simulink model "Bicycle_Posture_Regulator"  (R2024b)
settings: Solver=ode45  StartTime=0.0  StopTime=40  RelTol=1e-5
libraries: robotmobilelib x1, sim3dlib x1, sim3dautolib x1
settings Model: Creator=loren  LastModifiedBy=loren

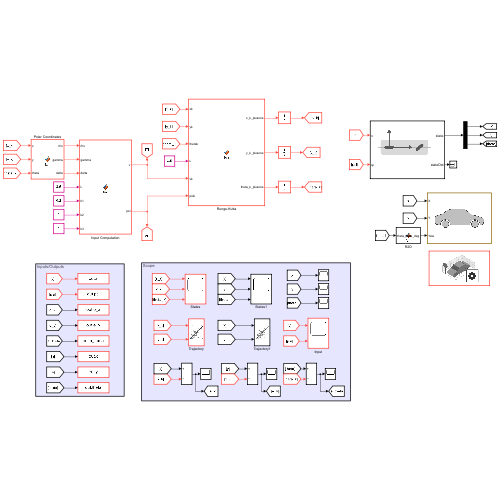
[thumbnail: Simulink's stored preview of the top-level diagram]
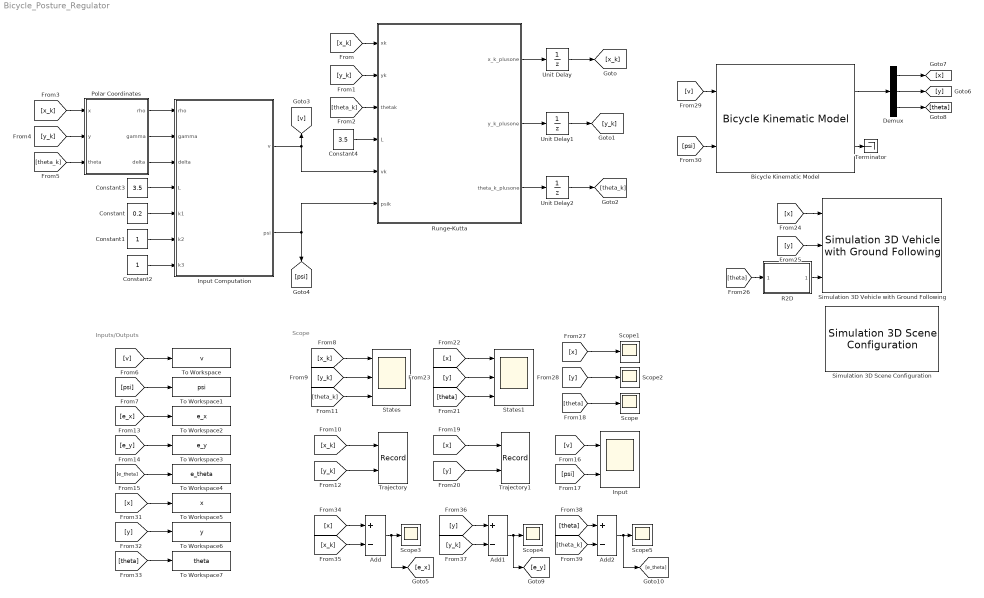
== system Bicycle_Posture_Regulator ==
  note: Scope
  note: Inputs/Outputs
  Add : Sum  Inputs=+-
  Add1 : Sum  Inputs=+-
  Add2 : Sum  Inputs=+-
  Bicycle Kinematic Model : robotmobilelib/Bicycle Kinematic Model  VehicleInputs=Vehicle Speed & Steering Angle  WheelBase=3.5  VehicleSpeedRange=[-inf inf]  MaxSteeringAngle=pi/3  InitialState=[-100; -50; pi/4]  SimulateUsing=Interpreted execution
  Constant : Constant  Value=0.2
  Constant1 : Constant
  Constant2 : Constant
  Constant3 : Constant  Value=3.5
  Constant4 : Constant  Value=3.5
  Demux : Demux  Outputs=3
  Input : Scope  NumInputPorts=2
  Input Computation : MATLAB Function  TreatAsAtomicUnit=on
  Polar Coordinates : MATLAB Function  TreatAsAtomicUnit=on
  R2D : MATLAB Function  TreatAsAtomicUnit=on
  Runge-Kutta : MATLAB Function  TreatAsAtomicUnit=on
  Scope{,1..5} (6 alike) : Scope
  Simulation 3D Scene Configuration : sim3dlib/Simulation 3D Scene Configuration  Priority=0  ProjectFormat=Default Scenes  SceneDesc=Parking lot  ProjectName=C:\Program Files\MATLAB\R2024b\toolbox\shared\sim3d_projects\automotive_project_windows\UE\WindowsNoEditor\VehicleSimulation.exe  ScenePath=/Game/Maps/HwStrght  EnableOpenDRIVE=off  vehTagList={'Custom';'Scene Origin';'SimulinkVehicle1'}  vehTag=SimulinkVehicle1  FreeCameraInitialTranslation=[0, 0, 0]  FreeCameraDefaultInitialTranslation=[-6, 0, 2]  FreeCameraInitialRotation=[0, 0, 0]  FreeCameraDefaultInitialRotation=[0, -15, 0]  OpVisEn=off  Ts=0.01  EnableWindow=on  EnableRemoteAccess=off  EnableWeather=off  SunAzimuth=90  SunAltitude=40.0  EnableGeospatialSun=off  Latitude=0  Longitude=0  Date=2023-01-01  Time=10:30:00  GeoTimeZone=-5.0  SunDaylightSaving=off  wind=1  clouds=10  EnableVolumetricClouds=off  CloudCoverage=0  CloudAltitude=6  fog=0  rain=0  RaindropsEffect=off  SnowDensity=0  EnableGeospatial=off  UseTrueOrigin=off  OriginHeight=200  OriginLatitude=40.744652  OriginLongitude=-73.988864  MapStyle=Aerial  AdditionalAssetIDs=[]  UseAdvancedSunSky=off  SolarTime=11  TimeZone=-5  Day=21  Month=9  Year=2022  UseDaylightSavingTime=on  DSTStartDay=10  DSTStartMonth=3  DSTEndDay=3  DSTEndMonth=11  DSTSwitchHour=2  sensorTag=MainCamera1  sensorId=1  sensorName=MainCamera1  mountLoc=Origin  offsetFlag=off  tmountOffset=[0, 0, 0]  rmountOffset=[0, 0, 0]  HorizontalResolution=1280  VerticalResolution=720  HorizontalFOV=60  mountPoint=[0 0 0]  mountOrientation=[0 0 0]  aMode=3  ID=1  GeoTrigger=Inactive
      settings: LibrarySourceBlock=drivingsim3d/Simulation 3D Scene Configuration
  Simulation 3D Vehicle with Ground Following : sim3dautolib/Simulation 3D Vehicle with Ground Following  Priority=-1  PassVehMesh=Muscle car  MeshPath=/MathWorksAutomotiveContent/Vehicles/Muscle/Meshes/SK_MuscleCar.SK_MuscleCar  TrackWidth=1.9  WheelBase=3  WheelRadius=0.35  VehColor=Red  InitialPos=[-100, -50, 0]  InitialRot=[0, 0, pi/4]  ActorName=SimulinkVehicle1  SampleTime=0.01  ActorType=SimulinkVehicle  ID=1  aMode=3  ActorTag=SimulinkVehicle1  CoordinateScheme=ISO  VehLightsControl=off  HeadlightColor=[ 1, 1, 1 ]  HighBeamIntensity=100000  LowBeamIntensity=60000  HighBeamConeAngle=70  LowBeamConeAngle=70  LeftHeadlightOrientation=[ 0, 0 ]  RightHeadlightOrientation=[ 0, 0 ]  BrakelightIntensity=500  ReverselightIntensity=500  SignallightIntensity=500  SignallightPeriod=1  SignalPulseWidth=50  TransformOutportEnabled=off
      settings: LibrarySourceBlock=drivingsim3d/Simulation 3D Vehicle with Ground Following
  States : Scope  NumInputPorts=3
  States1 : Scope  NumInputPorts=3
  Terminator : Terminator
  To Workspace : ToWorkspace  VariableName=v  SaveFormat=Timeseries  SampleTime=0.01
  To Workspace1 : ToWorkspace  VariableName=psi  SaveFormat=Timeseries  SampleTime=0.01
  To Workspace2 : ToWorkspace  VariableName=e_x  SaveFormat=Timeseries  SampleTime=0.01
  To Workspace3 : ToWorkspace  VariableName=e_y  SaveFormat=Timeseries  SampleTime=0.01
  To Workspace4 : ToWorkspace  VariableName=e_theta  SaveFormat=Timeseries  SampleTime=0.01
  To Workspace5 : ToWorkspace  VariableName=x  SaveFormat=Timeseries  SampleTime=0.01
  To Workspace6 : ToWorkspace  VariableName=y  SaveFormat=Timeseries  SampleTime=0.01
  To Workspace7 : ToWorkspace  VariableName=theta  SaveFormat=Timeseries  SampleTime=0.01
  Trajectory : Record  FileSettingsInternal="{\"entries\":[{\"content\":{\"excelSettings\":{\"content\":{},\"type\":\"Streamout.ExcelSettings\"}},\"type\":\"Streamout.FileSettingStorage\",\"uuid\":\"\"}],\"packageUris\":[\"http:\\/\\/schema.mathworks.com\\/mf0\\/streamout_blocks\\/R2020a\"],\"version\":\"1.0\"}"  Layout=[1 1]  SignalsInternal="{\"entries\":[{\"content\":{\"signals\":[{\"content\":{\"blockPath\":[],\"dimensions\":[1],\"domain\":\"\",\"lineColor\":\"#fe330a\",\"lineWidth\":2,\"port\":1,\"sid\":[\"\"],\"signalID\":1,\"signalName\":\"From10\"},\"type\":\"RecordBlkView.Signal\",\"uuid\":\"\"},{\"content\":{\"blockPath\":[],\"dimensions\":[1],\"domain\":\"\",\"lineColor\":\"#22b573\",\"lineWidth\":2,\"port\":2,\"sid\":[\"\"],\"signalID\":2,\"signalName\":\"From12\"},\"type\":\"RecordBlkView.Signal\",\"uuid\":\"\"}]},\"type\":\"RecordBlkView.InputSignals\",\"uuid\":\"\"}],\"packageUris\":[\"http:\\/\\/schema.mathworks.com\\/mf0\\/streamout_blocks\\/R2020a\"],\"version\":\"1.0\"}"  VisualizationBindings="{\"xyplotplugin\":{\"info\":[{\"series\":[],\"subplotID\":1}]}}"  CompatibilityTag=XY
  Trajectory1 : Record  FileSettingsInternal="{\"entries\":[{\"content\":{\"excelSettings\":{\"content\":{},\"type\":\"Streamout.ExcelSettings\"}},\"type\":\"Streamout.FileSettingStorage\",\"uuid\":\"\"}],\"packageUris\":[\"http:\\/\\/schema.mathworks.com\\/mf0\\/streamout_blocks\\/R2020a\"],\"version\":\"1.0\"}"  Layout=[1 1]  SignalsInternal="{\"entries\":[{\"content\":{\"signals\":[{\"content\":{\"blockPath\":[],\"dimensions\":[1],\"domain\":\"\",\"lineColor\":\"#a2142f\",\"plots\":[ 1 ],\"port\":1,\"sid\":[\"\"],\"signalID\":1,\"signalName\":\"From19\"},\"type\":\"RecordBlkView.Signal\",\"uuid\":\"\"},{\"content\":{\"blockPath\":[],\"dimensions\":[1],\"domain\":\"\",\"lineColor\":\"#139fff\",\"plots\":[ 1 ],\"port\":2,\"sid\":[\"\"],\"signalID\":2,\"signalName\":\"From20\"},\"type\":\"RecordBlkView.Signal\",\"uuid\":\"\"}]},\"type\":\"RecordBlkView.InputSignals\",\"uuid\":\"\"}],\"packageUris\":[\"http:\\/\\/schema.mathworks.com\\/mf0\\/streamout_blocks\\/R2020a\"],\"version\":\"1.0\"}"  VisualizationBindings="{\"xyplotplugin\":{\"info\":[{\"series\":[{\"bindingParametersList\":[{\"parameter\":\"X-Axis\",\"signalID\":1,\"signalName\":\"From19\"},{\"parameter\":\"Y-Axis\",\"signalID\":2,\"signalName\":\"From20\"}],\"seriesID\":0}],\"subplotID\":1}]}}"  CompatibilityTag=XY
  Unit Delay : UnitDelay  InitialCondition=-100  SampleTime=0.01  HasFrameUpgradeWarning=on
  Unit Delay1 : UnitDelay  InitialCondition=-50  SampleTime=0.01  HasFrameUpgradeWarning=on
  Unit Delay2 : UnitDelay  InitialCondition=pi/4  SampleTime=0.01  HasFrameUpgradeWarning=on
  wires:
  Constant/1 -> Input Computation/5(k1)
  Constant1/1 -> Input Computation/6(k2)
  Constant2/1 -> Input Computation/7(k3)
  Polar Coordinates/3(delta) -> Input Computation/3(delta)
  Polar Coordinates/2(gamma) -> Input Computation/2(gamma)
  Polar Coordinates/1(rho) -> Input Computation/1(rho)
  Input Computation/1(v) -> Runge-Kutta/5(vk), [v]
  Runge-Kutta/1(x_k_plusone) -> Unit Delay/1
  Runge-Kutta/2(y_k_plusone) -> Unit Delay1/1
  Runge-Kutta/3(theta_k_plusone) -> Unit Delay2/1
  Unit Delay/1 -> [x_k]
  Unit Delay1/1 -> [y_k]
  Unit Delay2/1 -> [theta_k]
  [x_k] -> Runge-Kutta/1(xk)
  [y_k] -> Runge-Kutta/2(yk)
  [theta_k] -> Runge-Kutta/3(thetak)
  [x_k] -> Polar Coordinates/1(x)
  [y_k] -> Polar Coordinates/2(y)
  [theta_k] -> Polar Coordinates/3(theta)
  [v] -> To Workspace/1
  [psi] -> To Workspace1/1
  [x_k] -> States/1
  [y_k] -> States/2
  [theta_k] -> States/3
  [x_k] -> Trajectory/1
  [y_k] -> Trajectory/2
  [e_x] -> To Workspace2/1
  [e_y] -> To Workspace3/1
  [e_theta] -> To Workspace4/1
  [v] -> Input/1
  [psi] -> Input/2
  Bicycle Kinematic Model/1 -> Demux/1
  Demux/2 -> [y]
  Demux/1 -> [x]
  Demux/3 -> [theta]
  Bicycle Kinematic Model/2 -> Terminator/1
  [x] -> Trajectory1/1
  [y] -> Trajectory1/2
  Input Computation/2(psi) -> [psi], Runge-Kutta/6(psik)
  [y] -> States1/2
  [x] -> States1/1
  [theta] -> States1/3
  [x] -> Simulation 3D Vehicle with Ground Following/1
  [y] -> Simulation 3D Vehicle with Ground Following/2
  R2D/1(theta_deg) -> Simulation 3D Vehicle with Ground Following/3
  [theta] -> R2D/1(theta_rad)
  [theta] -> Scope/1
  [x] -> Scope1/1
  [y] -> Scope2/1
  Constant3/1 -> Input Computation/4(L)
  [v] -> Bicycle Kinematic Model/1
  [psi] -> Bicycle Kinematic Model/2
  Constant4/1 -> Runge-Kutta/4(L)
  [theta] -> To Workspace7/1
  [y] -> To Workspace6/1
  [x] -> To Workspace5/1
  [x] -> Add/1
  [x_k] -> Add/2
  Add/1 -> [e_x], Scope3/1
  Add1/1 -> [e_y], Scope4/1
  [y] -> Add1/1
  [y_k] -> Add1/2
  Add2/1 -> [e_theta], Scope5/1
  [theta] -> Add2/1
  [theta_k] -> Add2/2

== matlab function Bicycle_Posture_Regulator/Input Computation ==
  data: rho input; gamma input; delta input; L input; v output; k1 input; k2 input; k3 input; psi output
function [v, psi] = fnc(rho, gamma, delta, L, k1, k2, k3)
    % Linear Velocity
    v = k1 * rho * cos(gamma);

    % Angular Velocity
    omega = k2 * gamma + k1 * sin(gamma) * cos(gamma) * (1 + k3 * (delta/gamma));

    % Steering Angle
    if abs(v) > 1e-6  % To avoid singularity
        psi = atan((omega * L) / v);
    else
        psi = 0;
    end

    % Maximum feasible value for psi
    psi_max = 60 * pi/180;  % ±60 gradi
    psi = max(-psi_max, min(psi_max, psi));
end

== matlab function Bicycle_Posture_Regulator/Polar Coordinates ==
  data: x input; rho output; y input; theta input; gamma output; delta output
function [rho, gamma, delta] = fcn(x, y, theta)

theta_d = -2/3*pi;

rho = sqrt(x^2 + y^2);
gamma = atan2(y,x) - theta + pi;
delta = gamma + theta + theta_d;

== matlab function Bicycle_Posture_Regulator/Runge-Kutta ==
  data: xk input; yk input; thetak input; L input; vk input; x_k_plusone output; psik input; y_k_plusone output; theta_k_plusone output
function [x_k_plusone, y_k_plusone, theta_k_plusone] = fcn(xk, yk, thetak, L, vk, psik)
    Ts = 0.01; % Sampling Time >0

    omegak = (vk / L) * tan(psik);

    x_k_plusone = xk + vk * Ts * cos(thetak + (omegak * Ts)/2);
    y_k_plusone = yk + vk * Ts * sin(thetak + (omegak * Ts)/2);
    theta_k_plusone = thetak + omegak * Ts;
end

== matlab function Bicycle_Posture_Regulator/R2D ==
  data: theta_rad input; theta_deg output
function theta_deg = fcn(theta_rad)

theta_deg = theta_rad*180/pi;
